simulink model "blockshemaotvorena"  (R2022b)
settings: Solver=VariableStepAuto  StartTime=0.0  StopTime=10.0  RelTol=1e-3
settings Model: Creator=mrxmi  LastModifiedBy=mrxmi

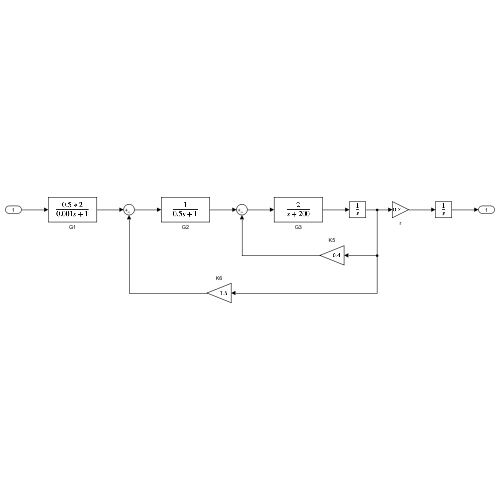
[thumbnail: Simulink's stored preview of the top-level diagram]
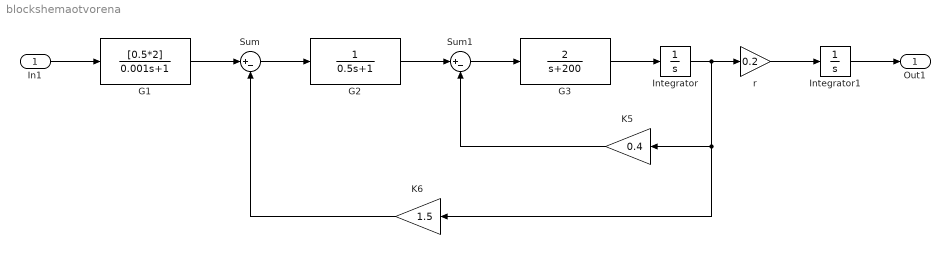
== system blockshemaotvorena ==
  In1 : Inport
  G1 : TransferFcn  Numerator=[0.5*2]  Denominator=[0.001 1]
  G2 : TransferFcn  Denominator=[0.5 1]
  G3 : TransferFcn  Numerator=[2]  Denominator=[1 200]
  Integrator : Integrator
  Integrator1 : Integrator
  K5 : Gain  Gain=0.4
  K6 : Gain  Gain=1.5
  Sum : Sum  Inputs=|+-
  Sum1 : Sum  Inputs=|+-
  r : Gain  Gain=0.2
  Out1 : Outport
  wires:
  Sum/1 -> G2/1
  In1/1 -> G1/1
  G1/1 -> Sum/1
  G2/1 -> Sum1/1
  Sum1/1 -> G3/1
  G3/1 -> Integrator/1
  Integrator/1 -> K6/1, K5/1, r/1
  r/1 -> Integrator1/1
  Integrator1/1 -> Out1/1
  K5/1 -> Sum1/2
  K6/1 -> Sum/2
